simulink model "sc_Regu_Study"  (R2016b)
settings: Solver=ode45  StartTime=0.0  StopTime=10.0  RelTol=1e-3  EnableMultiTasking=on
values from neighbouring files (symbols this model uses):
  denC = C.Denominator{1,1}    [Regu_study.m]
  denG = G.Denominator{1,1}    [Regu_study.m]
  ival_e = str2num(char(procede(2)))    [Regu_study.m]
  ival_ps = str2num(char(procede(8)))    [Regu_study.m]
  ival_pu = str2num(char(procede(5)))    [Regu_study.m]
  numC = C.Numerator{1,1}    [Regu_study.m]
  numG = G.Numerator{1,1}    [Regu_study.m]
  t_e = str2num(char(procede(1)))    [Regu_study.m]
  t_ps = str2num(char(procede(7)))    [Regu_study.m]
  t_pu = str2num(char(procede(4)))    [Regu_study.m]
  val_e = str2num(char(procede(3)))    [Regu_study.m]
  val_ps = str2num(char(procede(9)))    [Regu_study.m]
  val_pu = str2num(char(procede(6)))    [Regu_study.m]
settings Model: Creator=cmoniere  LastModifiedBy=Biscuit
settings DataIOCC: LimitDataPoints=on  SaveFormat=Array
settings OptimizationCC: LifeSpan=inf
settings DebuggingCC: SFUnexpectedBacktrackingDiag=warning  SFNoUnconditionalDefaultTransitionDiag=warning  SFExecutionAtInitializationDiag=none
settings HardwareCC: ProdBitPerPointer=32  ProdBitPerSizeT=32  ProdBitPerPtrDiffT=32  ProdLargestAtomicFloat=None  ProdIntDivRoundTo=Undefined  ProdEndianess=Unspecified  ProdWordSize=32  ProdHWDeviceType=32-bit Generic
settings ModelReferenceCC: PropagateSignalLabelsOutOfModel=off
settings GRTTargetCC: TargetLangStandard=C89/C90 (ANSI)  GeneratePreprocessorConditionals=Disable all
settings ConfigComp: CovMetricSettings=dw  CovHtmlReporting=on  CovSaveCumulativeToWorkspaceVar=on  CovSaveSingleToWorkspaceVar=on  CovExternalEMLEnable=off

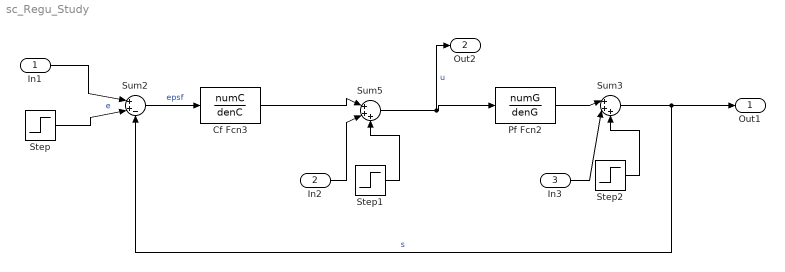
== system sc_Regu_Study ==
  In1 : Inport
  In2 : Inport  Port=2
  In3 : Inport  Port=3
  Cf Fcn3 : TransferFcn  Numerator=numC  Denominator=denC
  Pf Fcn2 : TransferFcn  Numerator=numG  Denominator=denG
  Step : Step  Time=t_e  Before=ival_e  After=val_e  SampleTime=0
  Step1 : Step  Time=t_pu  Before=ival_pu  After=val_pu  SampleTime=0
  Step2 : Step  Time=t_ps  Before=ival_ps  After=val_ps  SampleTime=0
  Sum2 : Sum  Inputs=|++-
  Sum3 : Sum  Inputs=|+++
  Sum5 : Sum  Inputs=|+++
  Out1 : Outport
  Out2 : Outport  Port=2
  wires:
  Sum2/1 -> Cf Fcn3/1  "epsf"
  In1/1 -> Sum2/1
  Sum3/1 -> Sum2/3, Out1/1  "s"
  Pf Fcn2/1 -> Sum3/1
  In3/1 -> Sum3/2
  In2/1 -> Sum5/2
  Cf Fcn3/1 -> Sum5/1
  Sum5/1 -> Out2/1, Pf Fcn2/1  "u"
  Step/1 -> Sum2/2  "e"
  Step1/1 -> Sum5/3
  Step2/1 -> Sum3/3
